simulink model "TST_CrCtl_StM"  (R2016b)
settings: Solver=FixedStepDiscrete  StartTime=0.0  StopTime=simTime  FixedStep=sampleTime  RelTol=1e-3
values from neighbouring files (symbols this model uses):
  testCase = 1    [initTST_CrCtl_StM_001.m]    (also in initTST_CrCtl_StM_002.m = 2)
libraries: simulink x31, UnitTest_Lib x18
(part 1 of 2)
settings Model: Creator=shiliwei  LastModifiedBy=shiliwei
settings DebuggingCC: SignalRangeChecking=error

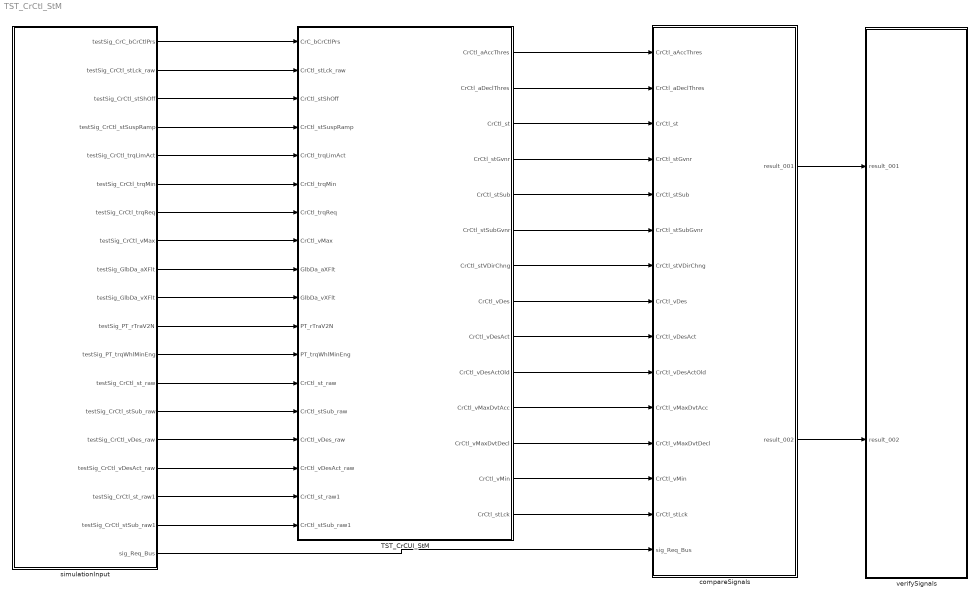
== system TST_CrCtl_StM ==
  TST_CrCUI_StM : Subsystem
  compareSignals : Subsystem
  simulationInput : Subsystem
  verifySignals : Subsystem
  wires:
  simulationInput/1(testSig_CrC_bCrCtlPrs) -> TST_CrCUI_StM/1(CrC_bCrCtlPrs)
  simulationInput/2(testSig_CrCtl_stLck_raw) -> TST_CrCUI_StM/2(CrCtl_stLck_raw)
  simulationInput/3(testSig_CrCtl_stShOff) -> TST_CrCUI_StM/3(CrCtl_stShOff)
  simulationInput/4(testSig_CrCtl_stSuspRamp) -> TST_CrCUI_StM/4(CrCtl_stSuspRamp)
  simulationInput/5(testSig_CrCtl_trqLimAct) -> TST_CrCUI_StM/5(CrCtl_trqLimAct)
  simulationInput/6(testSig_CrCtl_trqMin) -> TST_CrCUI_StM/6(CrCtl_trqMin)
  simulationInput/7(testSig_CrCtl_trqReq) -> TST_CrCUI_StM/7(CrCtl_trqReq)
  simulationInput/8(testSig_CrCtl_vMax) -> TST_CrCUI_StM/8(CrCtl_vMax)
  simulationInput/9(testSig_GlbDa_aXFlt) -> TST_CrCUI_StM/9(GlbDa_aXFlt)
  simulationInput/10(testSig_GlbDa_vXFlt) -> TST_CrCUI_StM/10(GlbDa_vXFlt)
  simulationInput/11(testSig_PT_rTraV2N) -> TST_CrCUI_StM/11(PT_rTraV2N)
  simulationInput/12(testSig_PT_trqWhlMinEng) -> TST_CrCUI_StM/12(PT_trqWhlMinEng)
  simulationInput/13(testSig_CrCtl_st_raw) -> TST_CrCUI_StM/13(CrCtl_st_raw)
  simulationInput/14(testSig_CrCtl_stSub_raw) -> TST_CrCUI_StM/14(CrCtl_stSub_raw)
  simulationInput/15(testSig_CrCtl_vDes_raw) -> TST_CrCUI_StM/15(CrCtl_vDes_raw)
  simulationInput/16(testSig_CrCtl_vDesAct_raw) -> TST_CrCUI_StM/16(CrCtl_vDesAct_raw)
  simulationInput/17(testSig_CrCtl_st_raw1) -> TST_CrCUI_StM/17(CrCtl_st_raw1)
  simulationInput/18(testSig_CrCtl_stSub_raw1) -> TST_CrCUI_StM/18(CrCtl_stSub_raw1)
  TST_CrCUI_StM/1(CrCtl_aAccThres) -> compareSignals/1(CrCtl_aAccThres)
  TST_CrCUI_StM/2(CrCtl_aDeclThres) -> compareSignals/2(CrCtl_aDeclThres)
  TST_CrCUI_StM/3(CrCtl_st) -> compareSignals/3(CrCtl_st)
  TST_CrCUI_StM/4(CrCtl_stGvnr) -> compareSignals/4(CrCtl_stGvnr)
  TST_CrCUI_StM/5(CrCtl_stSub) -> compareSignals/5(CrCtl_stSub)
  TST_CrCUI_StM/6(CrCtl_stSubGvnr) -> compareSignals/6(CrCtl_stSubGvnr)
  TST_CrCUI_StM/7(CrCtl_stVDirChng) -> compareSignals/7(CrCtl_stVDirChng)
  TST_CrCUI_StM/8(CrCtl_vDes) -> compareSignals/8(CrCtl_vDes)
  TST_CrCUI_StM/9(CrCtl_vDesAct) -> compareSignals/9(CrCtl_vDesAct)
  TST_CrCUI_StM/10(CrCtl_vDesActOld) -> compareSignals/10(CrCtl_vDesActOld)
  TST_CrCUI_StM/11(CrCtl_vMaxDvtAcc) -> compareSignals/11(CrCtl_vMaxDvtAcc)
  TST_CrCUI_StM/12(CrCtl_vMaxDvtDecl) -> compareSignals/12(CrCtl_vMaxDvtDecl)
  TST_CrCUI_StM/13(CrCtl_vMin) -> compareSignals/13(CrCtl_vMin)
  TST_CrCUI_StM/14(CrCtl_stLck) -> compareSignals/14(CrCtl_stLck)
  simulationInput/19(sig_Req_Bus) -> compareSignals/15(sig_Req_Bus)
  compareSignals/1(result_001) -> verifySignals/1(result_001)
  compareSignals/2(result_002) -> verifySignals/2(result_002)

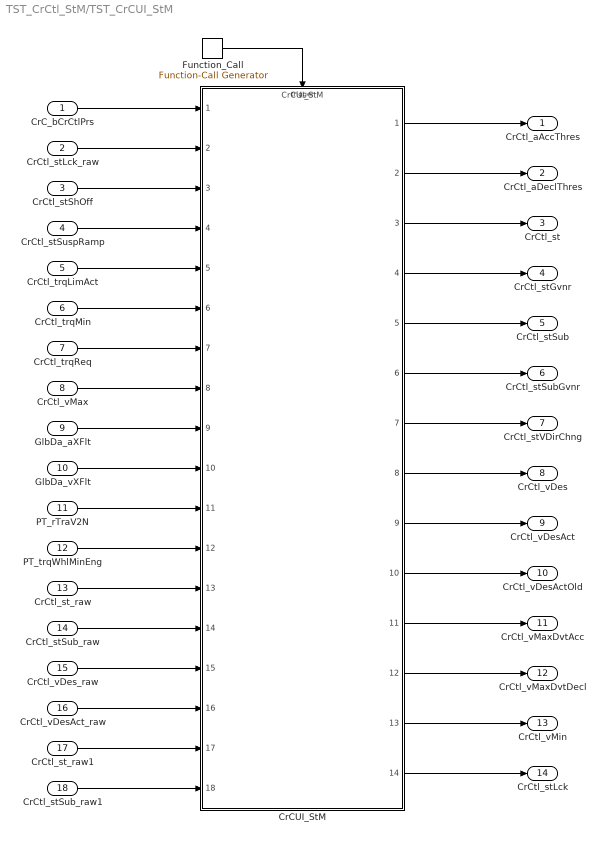
== system TST_CrCtl_StM/TST_CrCUI_StM ==
  CrC_bCrCtlPrs : Inport
  CrCtl_stLck_raw : Inport  Port=2
  CrCtl_stShOff : Inport  Port=3
  CrCtl_stSuspRamp : Inport  Port=4
  CrCtl_trqLimAct : Inport  Port=5
  CrCtl_trqMin : Inport  Port=6
  CrCtl_trqReq : Inport  Port=7
  CrCtl_vMax : Inport  Port=8
  GlbDa_aXFlt : Inport  Port=9
  GlbDa_vXFlt : Inport  Port=10
  PT_rTraV2N : Inport  Port=11
  PT_trqWhlMinEng : Inport  Port=12
  CrCtl_st_raw : Inport  Port=13
  CrCtl_stSub_raw : Inport  Port=14
  CrCtl_vDes_raw : Inport  Port=15
  CrCtl_vDesAct_raw : Inport  Port=16
  CrCtl_st_raw1 : Inport  Port=17
  CrCtl_stSub_raw1 : Inport  Port=18
  CrCUI_StM : ModelReference  ModelNameDialog=CrCUI_StM  SimulationMode=Normal  ModelReferenceVersion=1.63  TriggerPortName=function  TriggerPortTriggerType=function-call  TriggerPortStatesWhenEnabling=held
  Function_Call : simulink/Ports & Subsystems/Function-Call Generator  sample_time=sampleTime  numberOfIterations=1
  CrCtl_aAccThres : Outport
  CrCtl_aDeclThres : Outport  Port=2
  CrCtl_st : Outport  Port=3
  CrCtl_stGvnr : Outport  Port=4
  CrCtl_stSub : Outport  Port=5
  CrCtl_stSubGvnr : Outport  Port=6
  CrCtl_stVDirChng : Outport  Port=7
  CrCtl_vDes : Outport  Port=8
  CrCtl_vDesAct : Outport  Port=9
  CrCtl_vDesActOld : Outport  Port=10
  CrCtl_vMaxDvtAcc : Outport  Port=11
  CrCtl_vMaxDvtDecl : Outport  Port=12
  CrCtl_vMin : Outport  Port=13
  CrCtl_stLck : Outport  Port=14
  wires:
  Function_Call/1 -> CrCUI_StM/Trigger
  CrC_bCrCtlPrs/1 -> CrCUI_StM/1
  CrCtl_stLck_raw/1 -> CrCUI_StM/2
  CrCtl_stShOff/1 -> CrCUI_StM/3
  CrCtl_stSuspRamp/1 -> CrCUI_StM/4
  CrCtl_trqLimAct/1 -> CrCUI_StM/5
  CrCtl_trqMin/1 -> CrCUI_StM/6
  CrCtl_trqReq/1 -> CrCUI_StM/7
  CrCtl_vMax/1 -> CrCUI_StM/8
  GlbDa_aXFlt/1 -> CrCUI_StM/9
  GlbDa_vXFlt/1 -> CrCUI_StM/10
  PT_rTraV2N/1 -> CrCUI_StM/11
  PT_trqWhlMinEng/1 -> CrCUI_StM/12
  CrCtl_st_raw/1 -> CrCUI_StM/13
  CrCtl_stSub_raw/1 -> CrCUI_StM/14
  CrCtl_vDes_raw/1 -> CrCUI_StM/15
  CrCtl_vDesAct_raw/1 -> CrCUI_StM/16
  CrCtl_st_raw1/1 -> CrCUI_StM/17
  CrCtl_stSub_raw1/1 -> CrCUI_StM/18
  CrCUI_StM/1 -> CrCtl_aAccThres/1
  CrCUI_StM/2 -> CrCtl_aDeclThres/1
  CrCUI_StM/3 -> CrCtl_st/1
  CrCUI_StM/4 -> CrCtl_stGvnr/1
  CrCUI_StM/5 -> CrCtl_stSub/1
  CrCUI_StM/6 -> CrCtl_stSubGvnr/1
  CrCUI_StM/7 -> CrCtl_stVDirChng/1
  CrCUI_StM/8 -> CrCtl_vDes/1
  CrCUI_StM/9 -> CrCtl_vDesAct/1
  CrCUI_StM/10 -> CrCtl_vDesActOld/1
  CrCUI_StM/11 -> CrCtl_vMaxDvtAcc/1
  CrCUI_StM/12 -> CrCtl_vMaxDvtDecl/1
  CrCUI_StM/13 -> CrCtl_vMin/1
  CrCUI_StM/14 -> CrCtl_stLck/1

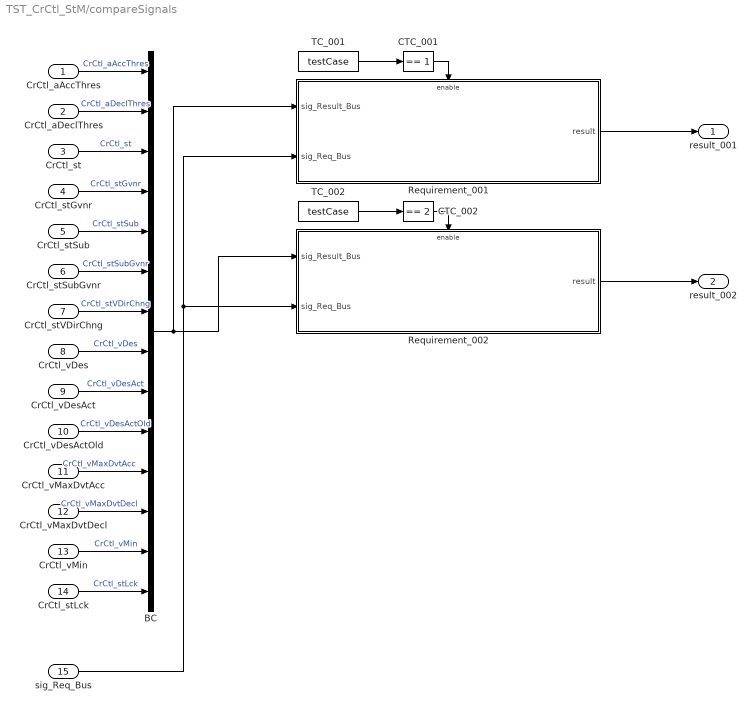
== system TST_CrCtl_StM/compareSignals ==
  CrCtl_aAccThres : Inport
  CrCtl_aDeclThres : Inport  Port=2
  CrCtl_st : Inport  Port=3
  CrCtl_stGvnr : Inport  Port=4
  CrCtl_stSub : Inport  Port=5
  CrCtl_stSubGvnr : Inport  Port=6
  CrCtl_stVDirChng : Inport  Port=7
  CrCtl_vDes : Inport  Port=8
  CrCtl_vDesAct : Inport  Port=9
  CrCtl_vDesActOld : Inport  Port=10
  CrCtl_vMaxDvtAcc : Inport  Port=11
  CrCtl_vMaxDvtDecl : Inport  Port=12
  CrCtl_vMin : Inport  Port=13
  CrCtl_stLck : Inport  Port=14
  sig_Req_Bus : Inport  Port=15
  BC : BusCreator  Inputs=14
  CTC_001 : simulink/Logic and Bit Operations/Compare To Constant  relop===  const=1  OutDataTypeStr=boolean
  CTC_002 : simulink/Logic and Bit Operations/Compare To Constant  relop===  const=2  OutDataTypeStr=boolean
  Requirement_001 : Subsystem
  Requirement_002 : Subsystem
  TC_001 : Constant  Value=testCase
  TC_002 : Constant  Value=testCase
  result_001 : Outport
  result_002 : Outport  Port=2
  wires:
  CrCtl_aAccThres/1 -> BC/1  "CrCtl_aAccThres"
  CrCtl_aDeclThres/1 -> BC/2  "CrCtl_aDeclThres"
  CrCtl_st/1 -> BC/3  "CrCtl_st"
  CrCtl_stGvnr/1 -> BC/4  "CrCtl_stGvnr"
  CrCtl_stSub/1 -> BC/5  "CrCtl_stSub"
  CrCtl_stSubGvnr/1 -> BC/6  "CrCtl_stSubGvnr"
  CrCtl_stVDirChng/1 -> BC/7  "CrCtl_stVDirChng"
  CrCtl_vDes/1 -> BC/8  "CrCtl_vDes"
  CrCtl_vDesAct/1 -> BC/9  "CrCtl_vDesAct"
  CrCtl_vDesActOld/1 -> BC/10  "CrCtl_vDesActOld"
  CrCtl_vMaxDvtAcc/1 -> BC/11  "CrCtl_vMaxDvtAcc"
  CrCtl_vMaxDvtDecl/1 -> BC/12  "CrCtl_vMaxDvtDecl"
  CrCtl_vMin/1 -> BC/13  "CrCtl_vMin"
  CrCtl_stLck/1 -> BC/14  "CrCtl_stLck"
  TC_001/1 -> CTC_001/1
  CTC_001/1 -> Requirement_001/Enable
  sig_Req_Bus/1 -> Requirement_001/2(sig_Req_Bus), Requirement_002/2(sig_Req_Bus)
  BC/1 -> Requirement_001/1(sig_Result_Bus), Requirement_002/1(sig_Result_Bus)
  Requirement_001/1(result) -> result_001/1
  TC_002/1 -> CTC_002/1
  CTC_002/1 -> Requirement_002/Enable
  Requirement_002/1(result) -> result_002/1

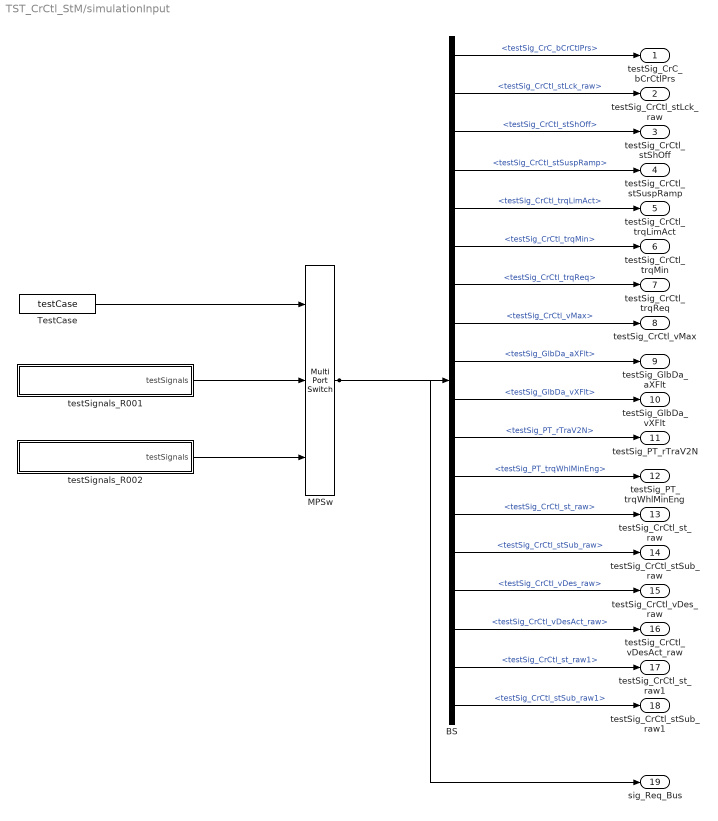
== system TST_CrCtl_StM/simulationInput ==
  BS : BusSelector  OutputSignals=testSig_CrC_bCrCtlPrs,testSig_CrCtl_stLck_raw,testSig_CrCtl_stShOff,testSig_CrCtl_stSuspRamp,testSig_CrCtl_trqLimAct,testSig_CrCtl_trqMin,testSig_CrCtl_trqReq,testSig_CrCtl_vMax,testSig_GlbDa_aXFlt,testSig_GlbDa_vXFlt,testSig_PT_rTraV2N,testSig_PT_trqWhlMinEng,testSig_CrCtl_st_raw,testSig_CrCtl_stSub_raw,testSig_CrCtl_vDes_raw,testSig_CrCtl_vDesAct_raw,testSig_CrCtl_st_raw1,testSig_CrCtl_stSub_raw1
  MPSw : MultiPortSwitch  Inputs=2  SaturateOnIntegerOverflow=on  InputSameDT=on
  TestCase : Constant  Value=testCase
  testSignals_R001 : Subsystem
  testSignals_R002 : Subsystem
  testSig_CrC_bCrCtlPrs : Outport
  testSig_CrCtl_stLck_raw : Outport  Port=2
  testSig_CrCtl_stShOff : Outport  Port=3
  testSig_CrCtl_stSuspRamp : Outport  Port=4
  testSig_CrCtl_trqLimAct : Outport  Port=5
  testSig_CrCtl_trqMin : Outport  Port=6
  testSig_CrCtl_trqReq : Outport  Port=7
  testSig_CrCtl_vMax : Outport  Port=8
  testSig_GlbDa_aXFlt : Outport  Port=9
  testSig_GlbDa_vXFlt : Outport  Port=10
  testSig_PT_rTraV2N : Outport  Port=11
  testSig_PT_trqWhlMinEng : Outport  Port=12
  testSig_CrCtl_st_raw : Outport  Port=13
  testSig_CrCtl_stSub_raw : Outport  Port=14
  testSig_CrCtl_vDes_raw : Outport  Port=15
  testSig_CrCtl_vDesAct_raw : Outport  Port=16
  testSig_CrCtl_st_raw1 : Outport  Port=17
  testSig_CrCtl_stSub_raw1 : Outport  Port=18
  sig_Req_Bus : Outport  Port=19
  wires:
  BS/1 -> testSig_CrC_bCrCtlPrs/1  "<testSig_CrC_bCrCtlPrs>"
  BS/2 -> testSig_CrCtl_stLck_raw/1  "<testSig_CrCtl_stLck_raw>"
  BS/3 -> testSig_CrCtl_stShOff/1  "<testSig_CrCtl_stShOff>"
  BS/4 -> testSig_CrCtl_stSuspRamp/1  "<testSig_CrCtl_stSuspRamp>"
  BS/5 -> testSig_CrCtl_trqLimAct/1  "<testSig_CrCtl_trqLimAct>"
  BS/6 -> testSig_CrCtl_trqMin/1  "<testSig_CrCtl_trqMin>"
  BS/7 -> testSig_CrCtl_trqReq/1  "<testSig_CrCtl_trqReq>"
  BS/8 -> testSig_CrCtl_vMax/1  "<testSig_CrCtl_vMax>"
  BS/9 -> testSig_GlbDa_aXFlt/1  "<testSig_GlbDa_aXFlt>"
  BS/10 -> testSig_GlbDa_vXFlt/1  "<testSig_GlbDa_vXFlt>"
  BS/11 -> testSig_PT_rTraV2N/1  "<testSig_PT_rTraV2N>"
  BS/12 -> testSig_PT_trqWhlMinEng/1  "<testSig_PT_trqWhlMinEng>"
  BS/13 -> testSig_CrCtl_st_raw/1  "<testSig_CrCtl_st_raw>"
  BS/14 -> testSig_CrCtl_stSub_raw/1  "<testSig_CrCtl_stSub_raw>"
  BS/15 -> testSig_CrCtl_vDes_raw/1  "<testSig_CrCtl_vDes_raw>"
  BS/16 -> testSig_CrCtl_vDesAct_raw/1  "<testSig_CrCtl_vDesAct_raw>"
  BS/17 -> testSig_CrCtl_st_raw1/1  "<testSig_CrCtl_st_raw1>"
  BS/18 -> testSig_CrCtl_stSub_raw1/1  "<testSig_CrCtl_stSub_raw1>"
  MPSw/1 -> BS/1, sig_Req_Bus/1
  TestCase/1 -> MPSw/1
  testSignals_R001/1(testSignals) -> MPSw/2
  testSignals_R002/1(testSignals) -> MPSw/3

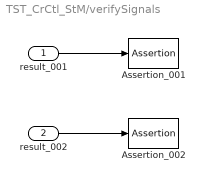
== system TST_CrCtl_StM/verifySignals ==
  result_001 : Inport
  result_002 : Inport  Port=2
  Assertion_001 : Assertion  Enabled=off
  Assertion_002 : Assertion  Enabled=off
  wires:
  result_001/1 -> Assertion_001/1
  result_002/1 -> Assertion_002/1

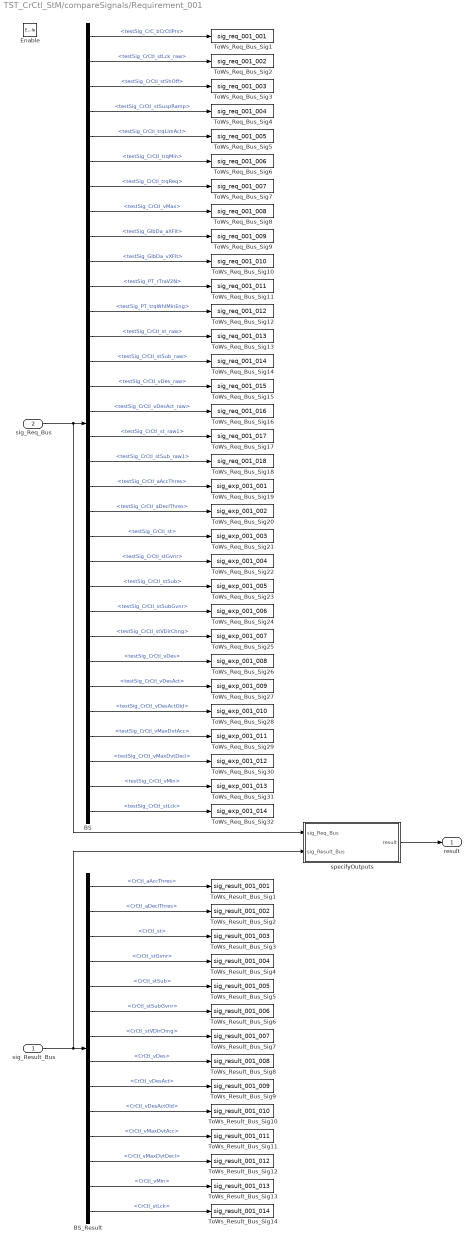
== system TST_CrCtl_StM/compareSignals/Requirement_001 ==
  sig_Result_Bus : Inport
  sig_Req_Bus : Inport  Port=2
  Enable : EnablePort
  BS : BusSelector  OutputSignals=testSig_CrC_bCrCtlPrs,testSig_CrCtl_stLck_raw,testSig_CrCtl_stShOff,testSig_CrCtl_stSuspRamp,testSig_CrCtl_trqLimAct,testSig_CrCtl_trqMin,testSig_CrCtl_trqReq,testSig_CrCtl_vMax,testSig_GlbDa_aXFlt,testSig_GlbDa_vXFlt,testSig_PT_rTraV2N,testSig_PT_trqWhlMinEng,testSig_CrCtl_st_raw,testSig_CrCtl_stSub_raw,testSig_CrCtl_vDes_raw,testSig_CrCtl_vDesAct_raw,testSig_CrCtl_st_raw1,testSig_CrCtl_stSub_raw1,testSig_CrCtl_aAccThres,testSig_CrCtl_aDeclThres,testSig_CrCtl_st,testSig_CrCtl_stGvnr,testSig_CrCtl_stSub,testSig_CrCtl_stSubGvnr,testSig_CrCtl_stVDirChng,testSig_CrCtl_vDes,testSig_CrCtl_vDesAct,testSig_CrCtl_vDesActOld,testSig_CrCtl_vMaxDvtAcc,testSig_CrCtl_vMaxDvtDecl,testSig_CrCtl_vMin,testSig_CrCtl_stLck
  BS_Result : BusSelector  OutputSignals=CrCtl_aAccThres,CrCtl_aDeclThres,CrCtl_st,CrCtl_stGvnr,CrCtl_stSub,CrCtl_stSubGvnr,CrCtl_stVDirChng,CrCtl_vDes,CrCtl_vDesAct,CrCtl_vDesActOld,CrCtl_vMaxDvtAcc,CrCtl_vMaxDvtDecl,CrCtl_vMin,CrCtl_stLck
  ToWs_Req_Bus_Sig1 : ToWorkspace  VariableName=sig_req_001_001  SaveFormat=Structure With Time
  ToWs_Req_Bus_Sig10 : ToWorkspace  VariableName=sig_req_001_010  SaveFormat=Structure With Time
  ToWs_Req_Bus_Sig11 : ToWorkspace  VariableName=sig_req_001_011  SaveFormat=Structure With Time
  ToWs_Req_Bus_Sig12 : ToWorkspace  VariableName=sig_req_001_012  SaveFormat=Structure With Time
  ToWs_Req_Bus_Sig13 : ToWorkspace  VariableName=sig_req_001_013  SaveFormat=Structure With Time
  ToWs_Req_Bus_Sig14 : ToWorkspace  VariableName=sig_req_001_014  SaveFormat=Structure With Time
  ToWs_Req_Bus_Sig15 : ToWorkspace  VariableName=sig_req_001_015  SaveFormat=Structure With Time
  ToWs_Req_Bus_Sig16 : ToWorkspace  VariableName=sig_req_001_016  SaveFormat=Structure With Time
  ToWs_Req_Bus_Sig17 : ToWorkspace  VariableName=sig_req_001_017  SaveFormat=Structure With Time
  ToWs_Req_Bus_Sig18 : ToWorkspace  VariableName=sig_req_001_018  SaveFormat=Structure With Time
  ToWs_Req_Bus_Sig19 : ToWorkspace  VariableName=sig_exp_001_001  SaveFormat=Structure With Time
  ToWs_Req_Bus_Sig2 : ToWorkspace  VariableName=sig_req_001_002  SaveFormat=Structure With Time
  ToWs_Req_Bus_Sig20 : ToWorkspace  VariableName=sig_exp_001_002  SaveFormat=Structure With Time
  ToWs_Req_Bus_Sig21 : ToWorkspace  VariableName=sig_exp_001_003  SaveFormat=Structure With Time
  ToWs_Req_Bus_Sig22 : ToWorkspace  VariableName=sig_exp_001_004  SaveFormat=Structure With Time
  ToWs_Req_Bus_Sig23 : ToWorkspace  VariableName=sig_exp_001_005  SaveFormat=Structure With Time
  ToWs_Req_Bus_Sig24 : ToWorkspace  VariableName=sig_exp_001_006  SaveFormat=Structure With Time
  ToWs_Req_Bus_Sig25 : ToWorkspace  VariableName=sig_exp_001_007  SaveFormat=Structure With Time
  ToWs_Req_Bus_Sig26 : ToWorkspace  VariableName=sig_exp_001_008  SaveFormat=Structure With Time
  ToWs_Req_Bus_Sig27 : ToWorkspace  VariableName=sig_exp_001_009  SaveFormat=Structure With Time
  ToWs_Req_Bus_Sig28 : ToWorkspace  VariableName=sig_exp_001_010  SaveFormat=Structure With Time
  ToWs_Req_Bus_Sig29 : ToWorkspace  VariableName=sig_exp_001_011  SaveFormat=Structure With Time
  ToWs_Req_Bus_Sig3 : ToWorkspace  VariableName=sig_req_001_003  SaveFormat=Structure With Time
  ToWs_Req_Bus_Sig30 : ToWorkspace  VariableName=sig_exp_001_012  SaveFormat=Structure With Time
  ToWs_Req_Bus_Sig31 : ToWorkspace  VariableName=sig_exp_001_013  SaveFormat=Structure With Time
  ToWs_Req_Bus_Sig32 : ToWorkspace  VariableName=sig_exp_001_014  SaveFormat=Structure With Time
  ToWs_Req_Bus_Sig4 : ToWorkspace  VariableName=sig_req_001_004  SaveFormat=Structure With Time
  ToWs_Req_Bus_Sig5 : ToWorkspace  VariableName=sig_req_001_005  SaveFormat=Structure With Time
  ToWs_Req_Bus_Sig6 : ToWorkspace  VariableName=sig_req_001_006  SaveFormat=Structure With Time
  ToWs_Req_Bus_Sig7 : ToWorkspace  VariableName=sig_req_001_007  SaveFormat=Structure With Time
  ToWs_Req_Bus_Sig8 : ToWorkspace  VariableName=sig_req_001_008  SaveFormat=Structure With Time
  ToWs_Req_Bus_Sig9 : ToWorkspace  VariableName=sig_req_001_009  SaveFormat=Structure With Time
  ToWs_Result_Bus_Sig1 : ToWorkspace  VariableName=sig_result_001_001  SaveFormat=Structure With Time
  ToWs_Result_Bus_Sig10 : ToWorkspace  VariableName=sig_result_001_010  SaveFormat=Structure With Time
  ToWs_Result_Bus_Sig11 : ToWorkspace  VariableName=sig_result_001_011  SaveFormat=Structure With Time
  ToWs_Result_Bus_Sig12 : ToWorkspace  VariableName=sig_result_001_012  SaveFormat=Structure With Time
  ToWs_Result_Bus_Sig13 : ToWorkspace  VariableName=sig_result_001_013  SaveFormat=Structure With Time
  ToWs_Result_Bus_Sig14 : ToWorkspace  VariableName=sig_result_001_014  SaveFormat=Structure With Time
  ToWs_Result_Bus_Sig2 : ToWorkspace  VariableName=sig_result_001_002  SaveFormat=Structure With Time
  ToWs_Result_Bus_Sig3 : ToWorkspace  VariableName=sig_result_001_003  SaveFormat=Structure With Time
  ToWs_Result_Bus_Sig4 : ToWorkspace  VariableName=sig_result_001_004  SaveFormat=Structure With Time
  ToWs_Result_Bus_Sig5 : ToWorkspace  VariableName=sig_result_001_005  SaveFormat=Structure With Time
  ToWs_Result_Bus_Sig6 : ToWorkspace  VariableName=sig_result_001_006  SaveFormat=Structure With Time
  ToWs_Result_Bus_Sig7 : ToWorkspace  VariableName=sig_result_001_007  SaveFormat=Structure With Time
  ToWs_Result_Bus_Sig8 : ToWorkspace  VariableName=sig_result_001_008  SaveFormat=Structure With Time
  ToWs_Result_Bus_Sig9 : ToWorkspace  VariableName=sig_result_001_009  SaveFormat=Structure With Time
  specifyOutputs : Subsystem
  result : Outport
  wires:
  sig_Req_Bus/1 -> BS/1, specifyOutputs/1(sig_Req_Bus)
  BS/1 -> ToWs_Req_Bus_Sig1/1  "<testSig_CrC_bCrCtlPrs>"
  BS/2 -> ToWs_Req_Bus_Sig2/1  "<testSig_CrCtl_stLck_raw>"
  BS/3 -> ToWs_Req_Bus_Sig3/1  "<testSig_CrCtl_stShOff>"
  BS/4 -> ToWs_Req_Bus_Sig4/1  "<testSig_CrCtl_stSuspRamp>"
  BS/5 -> ToWs_Req_Bus_Sig5/1  "<testSig_CrCtl_trqLimAct>"
  BS/6 -> ToWs_Req_Bus_Sig6/1  "<testSig_CrCtl_trqMin>"
  BS/7 -> ToWs_Req_Bus_Sig7/1  "<testSig_CrCtl_trqReq>"
  BS/8 -> ToWs_Req_Bus_Sig8/1  "<testSig_CrCtl_vMax>"
  BS/9 -> ToWs_Req_Bus_Sig9/1  "<testSig_GlbDa_aXFlt>"
  BS/10 -> ToWs_Req_Bus_Sig10/1  "<testSig_GlbDa_vXFlt>"
  BS/11 -> ToWs_Req_Bus_Sig11/1  "<testSig_PT_rTraV2N>"
  BS/12 -> ToWs_Req_Bus_Sig12/1  "<testSig_PT_trqWhlMinEng>"
  BS/13 -> ToWs_Req_Bus_Sig13/1  "<testSig_CrCtl_st_raw>"
  BS/14 -> ToWs_Req_Bus_Sig14/1  "<testSig_CrCtl_stSub_raw>"
  BS/15 -> ToWs_Req_Bus_Sig15/1  "<testSig_CrCtl_vDes_raw>"
  BS/16 -> ToWs_Req_Bus_Sig16/1  "<testSig_CrCtl_vDesAct_raw>"
  BS/17 -> ToWs_Req_Bus_Sig17/1  "<testSig_CrCtl_st_raw1>"
  BS/18 -> ToWs_Req_Bus_Sig18/1  "<testSig_CrCtl_stSub_raw1>"
  BS/19 -> ToWs_Req_Bus_Sig19/1  "<testSig_CrCtl_aAccThres>"
  BS/20 -> ToWs_Req_Bus_Sig20/1  "<testSig_CrCtl_aDeclThres>"
  BS/21 -> ToWs_Req_Bus_Sig21/1  "<testSig_CrCtl_st>"
  BS/22 -> ToWs_Req_Bus_Sig22/1  "<testSig_CrCtl_stGvnr>"
  BS/23 -> ToWs_Req_Bus_Sig23/1  "<testSig_CrCtl_stSub>"
  BS/24 -> ToWs_Req_Bus_Sig24/1  "<testSig_CrCtl_stSubGvnr>"
  BS/25 -> ToWs_Req_Bus_Sig25/1  "<testSig_CrCtl_stVDirChng>"
  BS/26 -> ToWs_Req_Bus_Sig26/1  "<testSig_CrCtl_vDes>"
  BS/27 -> ToWs_Req_Bus_Sig27/1  "<testSig_CrCtl_vDesAct>"
  BS/28 -> ToWs_Req_Bus_Sig28/1  "<testSig_CrCtl_vDesActOld>"
  BS/29 -> ToWs_Req_Bus_Sig29/1  "<testSig_CrCtl_vMaxDvtAcc>"
  BS/30 -> ToWs_Req_Bus_Sig30/1  "<testSig_CrCtl_vMaxDvtDecl>"
  BS/31 -> ToWs_Req_Bus_Sig31/1  "<testSig_CrCtl_vMin>"
  BS/32 -> ToWs_Req_Bus_Sig32/1  "<testSig_CrCtl_stLck>"
  sig_Result_Bus/1 -> BS_Result/1, specifyOutputs/2(sig_Result_Bus)
  BS_Result/1 -> ToWs_Result_Bus_Sig1/1  "<CrCtl_aAccThres>"
  BS_Result/2 -> ToWs_Result_Bus_Sig2/1  "<CrCtl_aDeclThres>"
  BS_Result/3 -> ToWs_Result_Bus_Sig3/1  "<CrCtl_st>"
  BS_Result/4 -> ToWs_Result_Bus_Sig4/1  "<CrCtl_stGvnr>"
  BS_Result/5 -> ToWs_Result_Bus_Sig5/1  "<CrCtl_stSub>"
  BS_Result/6 -> ToWs_Result_Bus_Sig6/1  "<CrCtl_stSubGvnr>"
  BS_Result/7 -> ToWs_Result_Bus_Sig7/1  "<CrCtl_stVDirChng>"
  BS_Result/8 -> ToWs_Result_Bus_Sig8/1  "<CrCtl_vDes>"
  BS_Result/9 -> ToWs_Result_Bus_Sig9/1  "<CrCtl_vDesAct>"
  BS_Result/10 -> ToWs_Result_Bus_Sig10/1  "<CrCtl_vDesActOld>"
  BS_Result/11 -> ToWs_Result_Bus_Sig11/1  "<CrCtl_vMaxDvtAcc>"
  BS_Result/12 -> ToWs_Result_Bus_Sig12/1  "<CrCtl_vMaxDvtDecl>"
  BS_Result/13 -> ToWs_Result_Bus_Sig13/1  "<CrCtl_vMin>"
  BS_Result/14 -> ToWs_Result_Bus_Sig14/1  "<CrCtl_stLck>"
  specifyOutputs/1(result) -> result/1

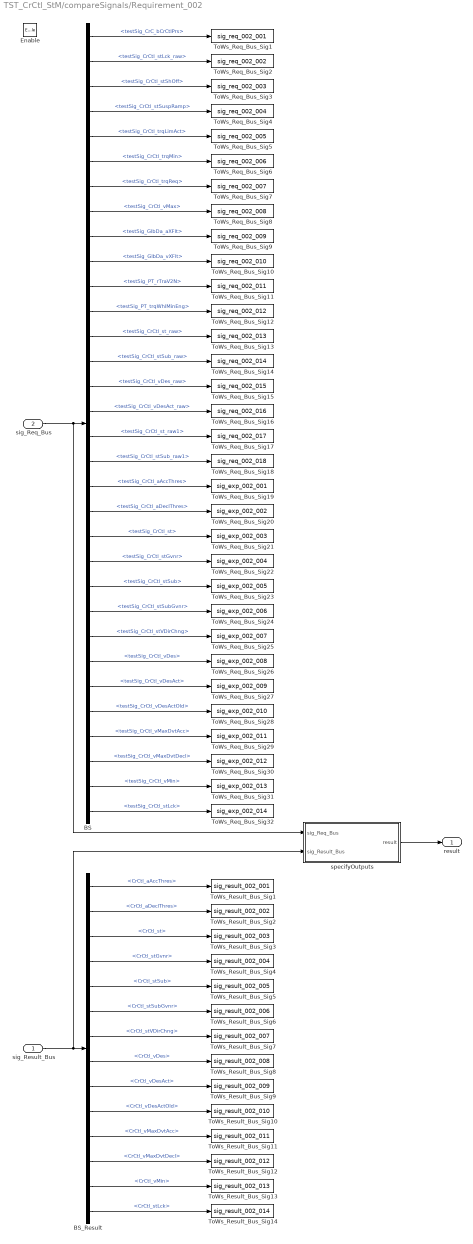
== system TST_CrCtl_StM/compareSignals/Requirement_002 ==
  sig_Result_Bus : Inport
  sig_Req_Bus : Inport  Port=2
  Enable : EnablePort
  BS : BusSelector  OutputSignals=testSig_CrC_bCrCtlPrs,testSig_CrCtl_stLck_raw,testSig_CrCtl_stShOff,testSig_CrCtl_stSuspRamp,testSig_CrCtl_trqLimAct,testSig_CrCtl_trqMin,testSig_CrCtl_trqReq,testSig_CrCtl_vMax,testSig_GlbDa_aXFlt,testSig_GlbDa_vXFlt,testSig_PT_rTraV2N,testSig_PT_trqWhlMinEng,testSig_CrCtl_st_raw,testSig_CrCtl_stSub_raw,testSig_CrCtl_vDes_raw,testSig_CrCtl_vDesAct_raw,testSig_CrCtl_st_raw1,testSig_CrCtl_stSub_raw1,testSig_CrCtl_aAccThres,testSig_CrCtl_aDeclThres,testSig_CrCtl_st,testSig_CrCtl_stGvnr,testSig_CrCtl_stSub,testSig_CrCtl_stSubGvnr,testSig_CrCtl_stVDirChng,testSig_CrCtl_vDes,testSig_CrCtl_vDesAct,testSig_CrCtl_vDesActOld,testSig_CrCtl_vMaxDvtAcc,testSig_CrCtl_vMaxDvtDecl,testSig_CrCtl_vMin,testSig_CrCtl_stLck
  BS_Result : BusSelector  OutputSignals=CrCtl_aAccThres,CrCtl_aDeclThres,CrCtl_st,CrCtl_stGvnr,CrCtl_stSub,CrCtl_stSubGvnr,CrCtl_stVDirChng,CrCtl_vDes,CrCtl_vDesAct,CrCtl_vDesActOld,CrCtl_vMaxDvtAcc,CrCtl_vMaxDvtDecl,CrCtl_vMin,CrCtl_stLck
  ToWs_Req_Bus_Sig1 : ToWorkspace  VariableName=sig_req_002_001  SaveFormat=Structure With Time
  ToWs_Req_Bus_Sig10 : ToWorkspace  VariableName=sig_req_002_010  SaveFormat=Structure With Time
  ToWs_Req_Bus_Sig11 : ToWorkspace  VariableName=sig_req_002_011  SaveFormat=Structure With Time
  ToWs_Req_Bus_Sig12 : ToWorkspace  VariableName=sig_req_002_012  SaveFormat=Structure With Time
  ToWs_Req_Bus_Sig13 : ToWorkspace  VariableName=sig_req_002_013  SaveFormat=Structure With Time
  ToWs_Req_Bus_Sig14 : ToWorkspace  VariableName=sig_req_002_014  SaveFormat=Structure With Time
  ToWs_Req_Bus_Sig15 : ToWorkspace  VariableName=sig_req_002_015  SaveFormat=Structure With Time
  ToWs_Req_Bus_Sig16 : ToWorkspace  VariableName=sig_req_002_016  SaveFormat=Structure With Time
  ToWs_Req_Bus_Sig17 : ToWorkspace  VariableName=sig_req_002_017  SaveFormat=Structure With Time
  ToWs_Req_Bus_Sig18 : ToWorkspace  VariableName=sig_req_002_018  SaveFormat=Structure With Time
  ToWs_Req_Bus_Sig19 : ToWorkspace  VariableName=sig_exp_002_001  SaveFormat=Structure With Time
  ToWs_Req_Bus_Sig2 : ToWorkspace  VariableName=sig_req_002_002  SaveFormat=Structure With Time
  ToWs_Req_Bus_Sig20 : ToWorkspace  VariableName=sig_exp_002_002  SaveFormat=Structure With Time
  ToWs_Req_Bus_Sig21 : ToWorkspace  VariableName=sig_exp_002_003  SaveFormat=Structure With Time
  ToWs_Req_Bus_Sig22 : ToWorkspace  VariableName=sig_exp_002_004  SaveFormat=Structure With Time
  ToWs_Req_Bus_Sig23 : ToWorkspace  VariableName=sig_exp_002_005  SaveFormat=Structure With Time
  ToWs_Req_Bus_Sig24 : ToWorkspace  VariableName=sig_exp_002_006  SaveFormat=Structure With Time
  ToWs_Req_Bus_Sig25 : ToWorkspace  VariableName=sig_exp_002_007  SaveFormat=Structure With Time
  ToWs_Req_Bus_Sig26 : ToWorkspace  VariableName=sig_exp_002_008  SaveFormat=Structure With Time
  ToWs_Req_Bus_Sig27 : ToWorkspace  VariableName=sig_exp_002_009  SaveFormat=Structure With Time
  ToWs_Req_Bus_Sig28 : ToWorkspace  VariableName=sig_exp_002_010  SaveFormat=Structure With Time
  ToWs_Req_Bus_Sig29 : ToWorkspace  VariableName=sig_exp_002_011  SaveFormat=Structure With Time
  ToWs_Req_Bus_Sig3 : ToWorkspace  VariableName=sig_req_002_003  SaveFormat=Structure With Time
  ToWs_Req_Bus_Sig30 : ToWorkspace  VariableName=sig_exp_002_012  SaveFormat=Structure With Time
  ToWs_Req_Bus_Sig31 : ToWorkspace  VariableName=sig_exp_002_013  SaveFormat=Structure With Time
  ToWs_Req_Bus_Sig32 : ToWorkspace  VariableName=sig_exp_002_014  SaveFormat=Structure With Time
  ToWs_Req_Bus_Sig4 : ToWorkspace  VariableName=sig_req_002_004  SaveFormat=Structure With Time
  ToWs_Req_Bus_Sig5 : ToWorkspace  VariableName=sig_req_002_005  SaveFormat=Structure With Time
  ToWs_Req_Bus_Sig6 : ToWorkspace  VariableName=sig_req_002_006  SaveFormat=Structure With Time
  ToWs_Req_Bus_Sig7 : ToWorkspace  VariableName=sig_req_002_007  SaveFormat=Structure With Time
  ToWs_Req_Bus_Sig8 : ToWorkspace  VariableName=sig_req_002_008  SaveFormat=Structure With Time
  ToWs_Req_Bus_Sig9 : ToWorkspace  VariableName=sig_req_002_009  SaveFormat=Structure With Time
  ToWs_Result_Bus_Sig1 : ToWorkspace  VariableName=sig_result_002_001  SaveFormat=Structure With Time
  ToWs_Result_Bus_Sig10 : ToWorkspace  VariableName=sig_result_002_010  SaveFormat=Structure With Time
  ToWs_Result_Bus_Sig11 : ToWorkspace  VariableName=sig_result_002_011  SaveFormat=Structure With Time
  ToWs_Result_Bus_Sig12 : ToWorkspace  VariableName=sig_result_002_012  SaveFormat=Structure With Time
  ToWs_Result_Bus_Sig13 : ToWorkspace  VariableName=sig_result_002_013  SaveFormat=Structure With Time
  ToWs_Result_Bus_Sig14 : ToWorkspace  VariableName=sig_result_002_014  SaveFormat=Structure With Time
  ToWs_Result_Bus_Sig2 : ToWorkspace  VariableName=sig_result_002_002  SaveFormat=Structure With Time
  ToWs_Result_Bus_Sig3 : ToWorkspace  VariableName=sig_result_002_003  SaveFormat=Structure With Time
  ToWs_Result_Bus_Sig4 : ToWorkspace  VariableName=sig_result_002_004  SaveFormat=Structure With Time
  ToWs_Result_Bus_Sig5 : ToWorkspace  VariableName=sig_result_002_005  SaveFormat=Structure With Time
  ToWs_Result_Bus_Sig6 : ToWorkspace  VariableName=sig_result_002_006  SaveFormat=Structure With Time
  ToWs_Result_Bus_Sig7 : ToWorkspace  VariableName=sig_result_002_007  SaveFormat=Structure With Time
  ToWs_Result_Bus_Sig8 : ToWorkspace  VariableName=sig_result_002_008  SaveFormat=Structure With Time
  ToWs_Result_Bus_Sig9 : ToWorkspace  VariableName=sig_result_002_009  SaveFormat=Structure With Time
  specifyOutputs : Subsystem
  result : Outport
  wires:
  sig_Req_Bus/1 -> BS/1, specifyOutputs/1(sig_Req_Bus)
  BS/1 -> ToWs_Req_Bus_Sig1/1  "<testSig_CrC_bCrCtlPrs>"
  BS/2 -> ToWs_Req_Bus_Sig2/1  "<testSig_CrCtl_stLck_raw>"
  BS/3 -> ToWs_Req_Bus_Sig3/1  "<testSig_CrCtl_stShOff>"
  BS/4 -> ToWs_Req_Bus_Sig4/1  "<testSig_CrCtl_stSuspRamp>"
  BS/5 -> ToWs_Req_Bus_Sig5/1  "<testSig_CrCtl_trqLimAct>"
  BS/6 -> ToWs_Req_Bus_Sig6/1  "<testSig_CrCtl_trqMin>"
  BS/7 -> ToWs_Req_Bus_Sig7/1  "<testSig_CrCtl_trqReq>"
  BS/8 -> ToWs_Req_Bus_Sig8/1  "<testSig_CrCtl_vMax>"
  BS/9 -> ToWs_Req_Bus_Sig9/1  "<testSig_GlbDa_aXFlt>"
  BS/10 -> ToWs_Req_Bus_Sig10/1  "<testSig_GlbDa_vXFlt>"
  BS/11 -> ToWs_Req_Bus_Sig11/1  "<testSig_PT_rTraV2N>"
  BS/12 -> ToWs_Req_Bus_Sig12/1  "<testSig_PT_trqWhlMinEng>"
  BS/13 -> ToWs_Req_Bus_Sig13/1  "<testSig_CrCtl_st_raw>"
  BS/14 -> ToWs_Req_Bus_Sig14/1  "<testSig_CrCtl_stSub_raw>"
  BS/15 -> ToWs_Req_Bus_Sig15/1  "<testSig_CrCtl_vDes_raw>"
  BS/16 -> ToWs_Req_Bus_Sig16/1  "<testSig_CrCtl_vDesAct_raw>"
  BS/17 -> ToWs_Req_Bus_Sig17/1  "<testSig_CrCtl_st_raw1>"
  BS/18 -> ToWs_Req_Bus_Sig18/1  "<testSig_CrCtl_stSub_raw1>"
  BS/19 -> ToWs_Req_Bus_Sig19/1  "<testSig_CrCtl_aAccThres>"
  BS/20 -> ToWs_Req_Bus_Sig20/1  "<testSig_CrCtl_aDeclThres>"
  BS/21 -> ToWs_Req_Bus_Sig21/1  "<testSig_CrCtl_st>"
  BS/22 -> ToWs_Req_Bus_Sig22/1  "<testSig_CrCtl_stGvnr>"
  BS/23 -> ToWs_Req_Bus_Sig23/1  "<testSig_CrCtl_stSub>"
  BS/24 -> ToWs_Req_Bus_Sig24/1  "<testSig_CrCtl_stSubGvnr>"
  BS/25 -> ToWs_Req_Bus_Sig25/1  "<testSig_CrCtl_stVDirChng>"
  BS/26 -> ToWs_Req_Bus_Sig26/1  "<testSig_CrCtl_vDes>"
  BS/27 -> ToWs_Req_Bus_Sig27/1  "<testSig_CrCtl_vDesAct>"
  BS/28 -> ToWs_Req_Bus_Sig28/1  "<testSig_CrCtl_vDesActOld>"
  BS/29 -> ToWs_Req_Bus_Sig29/1  "<testSig_CrCtl_vMaxDvtAcc>"
  BS/30 -> ToWs_Req_Bus_Sig30/1  "<testSig_CrCtl_vMaxDvtDecl>"
  BS/31 -> ToWs_Req_Bus_Sig31/1  "<testSig_CrCtl_vMin>"
  BS/32 -> ToWs_Req_Bus_Sig32/1  "<testSig_CrCtl_stLck>"
  sig_Result_Bus/1 -> BS_Result/1, specifyOutputs/2(sig_Result_Bus)
  BS_Result/1 -> ToWs_Result_Bus_Sig1/1  "<CrCtl_aAccThres>"
  BS_Result/2 -> ToWs_Result_Bus_Sig2/1  "<CrCtl_aDeclThres>"
  BS_Result/3 -> ToWs_Result_Bus_Sig3/1  "<CrCtl_st>"
  BS_Result/4 -> ToWs_Result_Bus_Sig4/1  "<CrCtl_stGvnr>"
  BS_Result/5 -> ToWs_Result_Bus_Sig5/1  "<CrCtl_stSub>"
  BS_Result/6 -> ToWs_Result_Bus_Sig6/1  "<CrCtl_stSubGvnr>"
  BS_Result/7 -> ToWs_Result_Bus_Sig7/1  "<CrCtl_stVDirChng>"
  BS_Result/8 -> ToWs_Result_Bus_Sig8/1  "<CrCtl_vDes>"
  BS_Result/9 -> ToWs_Result_Bus_Sig9/1  "<CrCtl_vDesAct>"
  BS_Result/10 -> ToWs_Result_Bus_Sig10/1  "<CrCtl_vDesActOld>"
  BS_Result/11 -> ToWs_Result_Bus_Sig11/1  "<CrCtl_vMaxDvtAcc>"
  BS_Result/12 -> ToWs_Result_Bus_Sig12/1  "<CrCtl_vMaxDvtDecl>"
  BS_Result/13 -> ToWs_Result_Bus_Sig13/1  "<CrCtl_vMin>"
  BS_Result/14 -> ToWs_Result_Bus_Sig14/1  "<CrCtl_stLck>"
  specifyOutputs/1(result) -> result/1

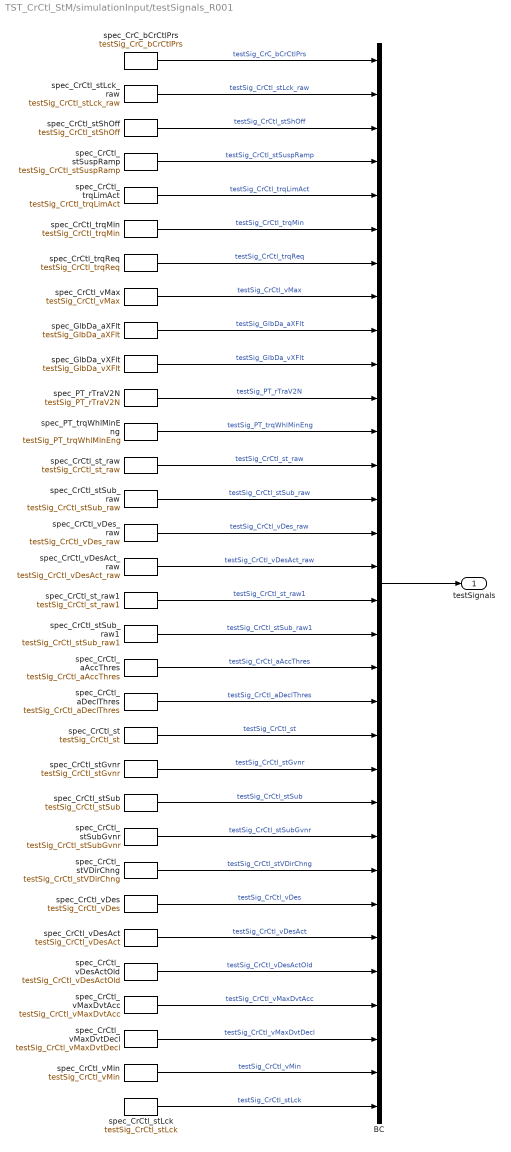
== system TST_CrCtl_StM/simulationInput/testSignals_R001 ==
  BC : BusCreator  Inputs=32
  spec_CrC_bCrCtlPrs : FromWorkspace  VariableName=testSig_CrC_bCrCtlPrs  Interpolate=off  OutputAfterFinalValue=Holding final value
  spec_CrCtl_aAccThres : FromWorkspace  VariableName=testSig_CrCtl_aAccThres  Interpolate=off  OutputAfterFinalValue=Holding final value
  spec_CrCtl_aDeclThres : FromWorkspace  VariableName=testSig_CrCtl_aDeclThres  Interpolate=off  OutputAfterFinalValue=Holding final value
  spec_CrCtl_st : FromWorkspace  VariableName=testSig_CrCtl_st  Interpolate=off  OutputAfterFinalValue=Holding final value
  spec_CrCtl_stGvnr : FromWorkspace  VariableName=testSig_CrCtl_stGvnr  Interpolate=off  OutputAfterFinalValue=Holding final value
  spec_CrCtl_stLck : FromWorkspace  VariableName=testSig_CrCtl_stLck  Interpolate=off  OutputAfterFinalValue=Holding final value
  spec_CrCtl_stLck_raw : FromWorkspace  VariableName=testSig_CrCtl_stLck_raw  Interpolate=off  OutputAfterFinalValue=Holding final value
  spec_CrCtl_stShOff : FromWorkspace  VariableName=testSig_CrCtl_stShOff  Interpolate=off  OutputAfterFinalValue=Holding final value
  spec_CrCtl_stSub : FromWorkspace  VariableName=testSig_CrCtl_stSub  Interpolate=off  OutputAfterFinalValue=Holding final value
  spec_CrCtl_stSubGvnr : FromWorkspace  VariableName=testSig_CrCtl_stSubGvnr  Interpolate=off  OutputAfterFinalValue=Holding final value
  spec_CrCtl_stSub_raw : FromWorkspace  VariableName=testSig_CrCtl_stSub_raw  Interpolate=off  OutputAfterFinalValue=Holding final value
  spec_CrCtl_stSub_raw1 : FromWorkspace  VariableName=testSig_CrCtl_stSub_raw1  Interpolate=off  OutputAfterFinalValue=Holding final value
  spec_CrCtl_stSuspRamp : FromWorkspace  VariableName=testSig_CrCtl_stSuspRamp  Interpolate=off  OutputAfterFinalValue=Holding final value
  spec_CrCtl_stVDirChng : FromWorkspace  VariableName=testSig_CrCtl_stVDirChng  Interpolate=off  OutputAfterFinalValue=Holding final value
  spec_CrCtl_st_raw : FromWorkspace  VariableName=testSig_CrCtl_st_raw  Interpolate=off  OutputAfterFinalValue=Holding final value
  spec_CrCtl_st_raw1 : FromWorkspace  VariableName=testSig_CrCtl_st_raw1  Interpolate=off  OutputAfterFinalValue=Holding final value
  spec_CrCtl_trqLimAct : FromWorkspace  VariableName=testSig_CrCtl_trqLimAct  Interpolate=off  OutputAfterFinalValue=Holding final value
  spec_CrCtl_trqMin : FromWorkspace  VariableName=testSig_CrCtl_trqMin  Interpolate=off  OutputAfterFinalValue=Holding final value
  spec_CrCtl_trqReq : FromWorkspace  VariableName=testSig_CrCtl_trqReq  Interpolate=off  OutputAfterFinalValue=Holding final value
  spec_CrCtl_vDes : FromWorkspace  VariableName=testSig_CrCtl_vDes  Interpolate=off  OutputAfterFinalValue=Holding final value
  spec_CrCtl_vDesAct : FromWorkspace  VariableName=testSig_CrCtl_vDesAct  Interpolate=off  OutputAfterFinalValue=Holding final value
  spec_CrCtl_vDesActOld : FromWorkspace  VariableName=testSig_CrCtl_vDesActOld  Interpolate=off  OutputAfterFinalValue=Holding final value
  spec_CrCtl_vDesAct_raw : FromWorkspace  VariableName=testSig_CrCtl_vDesAct_raw  Interpolate=off  OutputAfterFinalValue=Holding final value
  spec_CrCtl_vDes_raw : FromWorkspace  VariableName=testSig_CrCtl_vDes_raw  Interpolate=off  OutputAfterFinalValue=Holding final value
  spec_CrCtl_vMax : FromWorkspace  VariableName=testSig_CrCtl_vMax  Interpolate=off  OutputAfterFinalValue=Holding final value
  spec_CrCtl_vMaxDvtAcc : FromWorkspace  VariableName=testSig_CrCtl_vMaxDvtAcc  Interpolate=off  OutputAfterFinalValue=Holding final value
  spec_CrCtl_vMaxDvtDecl : FromWorkspace  VariableName=testSig_CrCtl_vMaxDvtDecl  Interpolate=off  OutputAfterFinalValue=Holding final value
  spec_CrCtl_vMin : FromWorkspace  VariableName=testSig_CrCtl_vMin  Interpolate=off  OutputAfterFinalValue=Holding final value
  spec_GlbDa_aXFlt : FromWorkspace  VariableName=testSig_GlbDa_aXFlt  Interpolate=off  OutputAfterFinalValue=Holding final value
  spec_GlbDa_vXFlt : FromWorkspace  VariableName=testSig_GlbDa_vXFlt  Interpolate=off  OutputAfterFinalValue=Holding final value
  spec_PT_rTraV2N : FromWorkspace  VariableName=testSig_PT_rTraV2N  Interpolate=off  OutputAfterFinalValue=Holding final value
  spec_PT_trqWhlMinEng : FromWorkspace  VariableName=testSig_PT_trqWhlMinEng  Interpolate=off  OutputAfterFinalValue=Holding final value
  testSignals : Outport
  wires:
  BC/1 -> testSignals/1
  spec_CrC_bCrCtlPrs/1 -> BC/1  "testSig_CrC_bCrCtlPrs"
  spec_CrCtl_stLck_raw/1 -> BC/2  "testSig_CrCtl_stLck_raw"
  spec_CrCtl_stShOff/1 -> BC/3  "testSig_CrCtl_stShOff"
  spec_CrCtl_stSuspRamp/1 -> BC/4  "testSig_CrCtl_stSuspRamp"
  spec_CrCtl_trqLimAct/1 -> BC/5  "testSig_CrCtl_trqLimAct"
  spec_CrCtl_trqMin/1 -> BC/6  "testSig_CrCtl_trqMin"
  spec_CrCtl_trqReq/1 -> BC/7  "testSig_CrCtl_trqReq"
  spec_CrCtl_vMax/1 -> BC/8  "testSig_CrCtl_vMax"
  spec_GlbDa_aXFlt/1 -> BC/9  "testSig_GlbDa_aXFlt"
  spec_GlbDa_vXFlt/1 -> BC/10  "testSig_GlbDa_vXFlt"
  spec_PT_rTraV2N/1 -> BC/11  "testSig_PT_rTraV2N"
  spec_PT_trqWhlMinEng/1 -> BC/12  "testSig_PT_trqWhlMinEng"
  spec_CrCtl_st_raw/1 -> BC/13  "testSig_CrCtl_st_raw"
  spec_CrCtl_stSub_raw/1 -> BC/14  "testSig_CrCtl_stSub_raw"
  spec_CrCtl_vDes_raw/1 -> BC/15  "testSig_CrCtl_vDes_raw"
  spec_CrCtl_vDesAct_raw/1 -> BC/16  "testSig_CrCtl_vDesAct_raw"
  spec_CrCtl_st_raw1/1 -> BC/17  "testSig_CrCtl_st_raw1"
  spec_CrCtl_stSub_raw1/1 -> BC/18  "testSig_CrCtl_stSub_raw1"
  spec_CrCtl_aAccThres/1 -> BC/19  "testSig_CrCtl_aAccThres"
  spec_CrCtl_aDeclThres/1 -> BC/20  "testSig_CrCtl_aDeclThres"
  spec_CrCtl_st/1 -> BC/21  "testSig_CrCtl_st"
  spec_CrCtl_stGvnr/1 -> BC/22  "testSig_CrCtl_stGvnr"
  spec_CrCtl_stSub/1 -> BC/23  "testSig_CrCtl_stSub"
  spec_CrCtl_stSubGvnr/1 -> BC/24  "testSig_CrCtl_stSubGvnr"
  spec_CrCtl_stVDirChng/1 -> BC/25  "testSig_CrCtl_stVDirChng"
  spec_CrCtl_vDes/1 -> BC/26  "testSig_CrCtl_vDes"
  spec_CrCtl_vDesAct/1 -> BC/27  "testSig_CrCtl_vDesAct"
  spec_CrCtl_vDesActOld/1 -> BC/28  "testSig_CrCtl_vDesActOld"
  spec_CrCtl_vMaxDvtAcc/1 -> BC/29  "testSig_CrCtl_vMaxDvtAcc"
  spec_CrCtl_vMaxDvtDecl/1 -> BC/30  "testSig_CrCtl_vMaxDvtDecl"
  spec_CrCtl_vMin/1 -> BC/31  "testSig_CrCtl_vMin"
  spec_CrCtl_stLck/1 -> BC/32  "testSig_CrCtl_stLck"

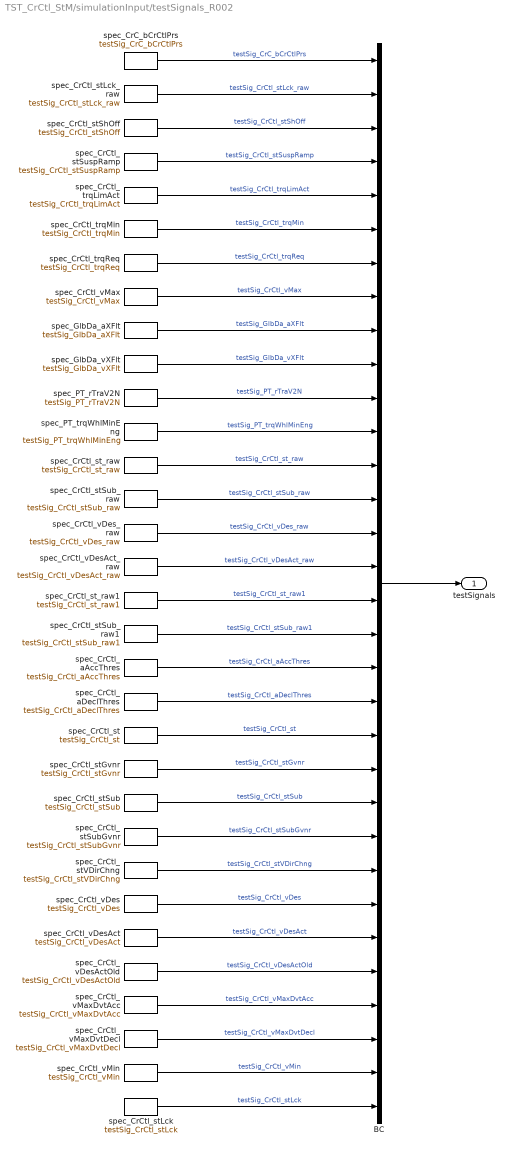
== system TST_CrCtl_StM/simulationInput/testSignals_R002 ==
  BC : BusCreator  Inputs=32
  spec_CrC_bCrCtlPrs : FromWorkspace  VariableName=testSig_CrC_bCrCtlPrs  Interpolate=off  OutputAfterFinalValue=Holding final value
  spec_CrCtl_aAccThres : FromWorkspace  VariableName=testSig_CrCtl_aAccThres  Interpolate=off  OutputAfterFinalValue=Holding final value
  spec_CrCtl_aDeclThres : FromWorkspace  VariableName=testSig_CrCtl_aDeclThres  Interpolate=off  OutputAfterFinalValue=Holding final value
  spec_CrCtl_st : FromWorkspace  VariableName=testSig_CrCtl_st  Interpolate=off  OutputAfterFinalValue=Holding final value
  spec_CrCtl_stGvnr : FromWorkspace  VariableName=testSig_CrCtl_stGvnr  Interpolate=off  OutputAfterFinalValue=Holding final value
  spec_CrCtl_stLck : FromWorkspace  VariableName=testSig_CrCtl_stLck  Interpolate=off  OutputAfterFinalValue=Holding final value
  spec_CrCtl_stLck_raw : FromWorkspace  VariableName=testSig_CrCtl_stLck_raw  Interpolate=off  OutputAfterFinalValue=Holding final value
  spec_CrCtl_stShOff : FromWorkspace  VariableName=testSig_CrCtl_stShOff  Interpolate=off  OutputAfterFinalValue=Holding final value
  spec_CrCtl_stSub : FromWorkspace  VariableName=testSig_CrCtl_stSub  Interpolate=off  OutputAfterFinalValue=Holding final value
  spec_CrCtl_stSubGvnr : FromWorkspace  VariableName=testSig_CrCtl_stSubGvnr  Interpolate=off  OutputAfterFinalValue=Holding final value
  spec_CrCtl_stSub_raw : FromWorkspace  VariableName=testSig_CrCtl_stSub_raw  Interpolate=off  OutputAfterFinalValue=Holding final value
  spec_CrCtl_stSub_raw1 : FromWorkspace  VariableName=testSig_CrCtl_stSub_raw1  Interpolate=off  OutputAfterFinalValue=Holding final value
  spec_CrCtl_stSuspRamp : FromWorkspace  VariableName=testSig_CrCtl_stSuspRamp  Interpolate=off  OutputAfterFinalValue=Holding final value
  spec_CrCtl_stVDirChng : FromWorkspace  VariableName=testSig_CrCtl_stVDirChng  Interpolate=off  OutputAfterFinalValue=Holding final value
  spec_CrCtl_st_raw : FromWorkspace  VariableName=testSig_CrCtl_st_raw  Interpolate=off  OutputAfterFinalValue=Holding final value
  spec_CrCtl_st_raw1 : FromWorkspace  VariableName=testSig_CrCtl_st_raw1  Interpolate=off  OutputAfterFinalValue=Holding final value
  spec_CrCtl_trqLimAct : FromWorkspace  VariableName=testSig_CrCtl_trqLimAct  Interpolate=off  OutputAfterFinalValue=Holding final value
  spec_CrCtl_trqMin : FromWorkspace  VariableName=testSig_CrCtl_trqMin  Interpolate=off  OutputAfterFinalValue=Holding final value
  spec_CrCtl_trqReq : FromWorkspace  VariableName=testSig_CrCtl_trqReq  Interpolate=off  OutputAfterFinalValue=Holding final value
  spec_CrCtl_vDes : FromWorkspace  VariableName=testSig_CrCtl_vDes  Interpolate=off  OutputAfterFinalValue=Holding final value
  spec_CrCtl_vDesAct : FromWorkspace  VariableName=testSig_CrCtl_vDesAct  Interpolate=off  OutputAfterFinalValue=Holding final value
  spec_CrCtl_vDesActOld : FromWorkspace  VariableName=testSig_CrCtl_vDesActOld  Interpolate=off  OutputAfterFinalValue=Holding final value
  spec_CrCtl_vDesAct_raw : FromWorkspace  VariableName=testSig_CrCtl_vDesAct_raw  Interpolate=off  OutputAfterFinalValue=Holding final value
  spec_CrCtl_vDes_raw : FromWorkspace  VariableName=testSig_CrCtl_vDes_raw  Interpolate=off  OutputAfterFinalValue=Holding final value
  spec_CrCtl_vMax : FromWorkspace  VariableName=testSig_CrCtl_vMax  Interpolate=off  OutputAfterFinalValue=Holding final value
  spec_CrCtl_vMaxDvtAcc : FromWorkspace  VariableName=testSig_CrCtl_vMaxDvtAcc  Interpolate=off  OutputAfterFinalValue=Holding final value
  spec_CrCtl_vMaxDvtDecl : FromWorkspace  VariableName=testSig_CrCtl_vMaxDvtDecl  Interpolate=off  OutputAfterFinalValue=Holding final value
  spec_CrCtl_vMin : FromWorkspace  VariableName=testSig_CrCtl_vMin  Interpolate=off  OutputAfterFinalValue=Holding final value
  spec_GlbDa_aXFlt : FromWorkspace  VariableName=testSig_GlbDa_aXFlt  Interpolate=off  OutputAfterFinalValue=Holding final value
  spec_GlbDa_vXFlt : FromWorkspace  VariableName=testSig_GlbDa_vXFlt  Interpolate=off  OutputAfterFinalValue=Holding final value
  spec_PT_rTraV2N : FromWorkspace  VariableName=testSig_PT_rTraV2N  Interpolate=off  OutputAfterFinalValue=Holding final value
  spec_PT_trqWhlMinEng : FromWorkspace  VariableName=testSig_PT_trqWhlMinEng  Interpolate=off  OutputAfterFinalValue=Holding final value
  testSignals : Outport
  wires:
  BC/1 -> testSignals/1
  spec_CrC_bCrCtlPrs/1 -> BC/1  "testSig_CrC_bCrCtlPrs"
  spec_CrCtl_stLck_raw/1 -> BC/2  "testSig_CrCtl_stLck_raw"
  spec_CrCtl_stShOff/1 -> BC/3  "testSig_CrCtl_stShOff"
  spec_CrCtl_stSuspRamp/1 -> BC/4  "testSig_CrCtl_stSuspRamp"
  spec_CrCtl_trqLimAct/1 -> BC/5  "testSig_CrCtl_trqLimAct"
  spec_CrCtl_trqMin/1 -> BC/6  "testSig_CrCtl_trqMin"
  spec_CrCtl_trqReq/1 -> BC/7  "testSig_CrCtl_trqReq"
  spec_CrCtl_vMax/1 -> BC/8  "testSig_CrCtl_vMax"
  spec_GlbDa_aXFlt/1 -> BC/9  "testSig_GlbDa_aXFlt"
  spec_GlbDa_vXFlt/1 -> BC/10  "testSig_GlbDa_vXFlt"
  spec_PT_rTraV2N/1 -> BC/11  "testSig_PT_rTraV2N"
  spec_PT_trqWhlMinEng/1 -> BC/12  "testSig_PT_trqWhlMinEng"
  spec_CrCtl_st_raw/1 -> BC/13  "testSig_CrCtl_st_raw"
  spec_CrCtl_stSub_raw/1 -> BC/14  "testSig_CrCtl_stSub_raw"
  spec_CrCtl_vDes_raw/1 -> BC/15  "testSig_CrCtl_vDes_raw"
  spec_CrCtl_vDesAct_raw/1 -> BC/16  "testSig_CrCtl_vDesAct_raw"
  spec_CrCtl_st_raw1/1 -> BC/17  "testSig_CrCtl_st_raw1"
  spec_CrCtl_stSub_raw1/1 -> BC/18  "testSig_CrCtl_stSub_raw1"
  spec_CrCtl_aAccThres/1 -> BC/19  "testSig_CrCtl_aAccThres"
  spec_CrCtl_aDeclThres/1 -> BC/20  "testSig_CrCtl_aDeclThres"
  spec_CrCtl_st/1 -> BC/21  "testSig_CrCtl_st"
  spec_CrCtl_stGvnr/1 -> BC/22  "testSig_CrCtl_stGvnr"
  spec_CrCtl_stSub/1 -> BC/23  "testSig_CrCtl_stSub"
  spec_CrCtl_stSubGvnr/1 -> BC/24  "testSig_CrCtl_stSubGvnr"
  spec_CrCtl_stVDirChng/1 -> BC/25  "testSig_CrCtl_stVDirChng"
  spec_CrCtl_vDes/1 -> BC/26  "testSig_CrCtl_vDes"
  spec_CrCtl_vDesAct/1 -> BC/27  "testSig_CrCtl_vDesAct"
  spec_CrCtl_vDesActOld/1 -> BC/28  "testSig_CrCtl_vDesActOld"
  spec_CrCtl_vMaxDvtAcc/1 -> BC/29  "testSig_CrCtl_vMaxDvtAcc"
  spec_CrCtl_vMaxDvtDecl/1 -> BC/30  "testSig_CrCtl_vMaxDvtDecl"
  spec_CrCtl_vMin/1 -> BC/31  "testSig_CrCtl_vMin"
  spec_CrCtl_stLck/1 -> BC/32  "testSig_CrCtl_stLck"

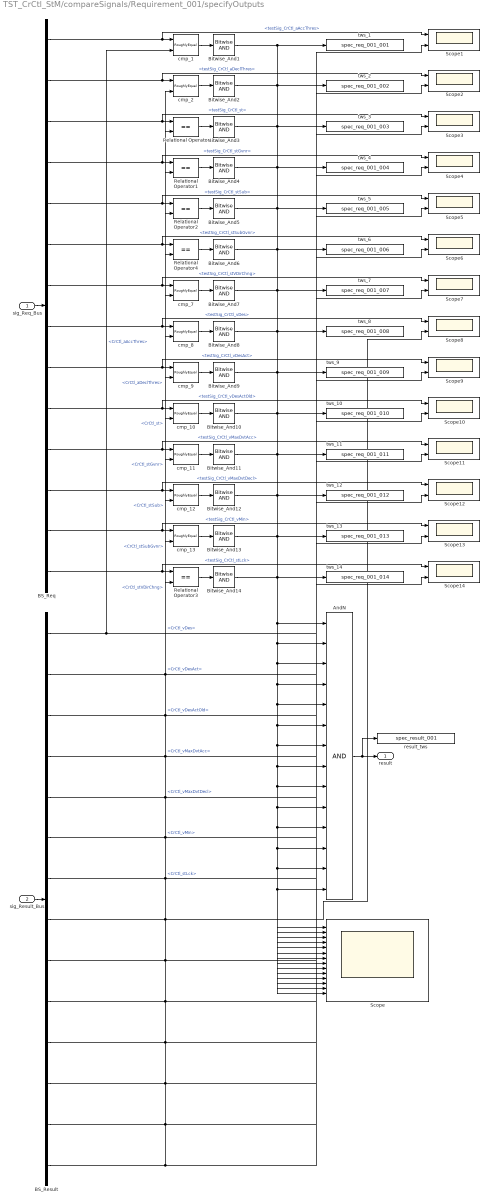
== system TST_CrCtl_StM/compareSignals/Requirement_001/specifyOutputs ==
  sig_Req_Bus : Inport
  sig_Result_Bus : Inport  Port=2
  AndN : Logic  Inputs=14
  BS_Req : BusSelector  OutputSignals=testSig_CrCtl_aAccThres,testSig_CrCtl_aDeclThres,testSig_CrCtl_st,testSig_CrCtl_stGvnr,testSig_CrCtl_stSub,testSig_CrCtl_stSubGvnr,testSig_CrCtl_stVDirChng,testSig_CrCtl_vDes,testSig_CrCtl_vDesAct,testSig_CrCtl_vDesActOld,testSig_CrCtl_vMaxDvtAcc,testSig_CrCtl_vMaxDvtDecl,testSig_CrCtl_vMin,testSig_CrCtl_stLck
  BS_Result : BusSelector  OutputSignals=CrCtl_aAccThres,CrCtl_aDeclThres,CrCtl_st,CrCtl_stGvnr,CrCtl_stSub,CrCtl_stSubGvnr,CrCtl_stVDirChng,CrCtl_vDes,CrCtl_vDesAct,CrCtl_vDesActOld,CrCtl_vMaxDvtAcc,CrCtl_vMaxDvtDecl,CrCtl_vMin,CrCtl_stLck
  Bitwise_And{1..14} (14 alike) : simulink/Logic and Bit Operations/Bitwise Operator  logicop=AND  UseBitMask=off  BitMask=bin2dec('11011001')  BitMaskRealWorld=Stored Integer
  Relational Operator{,1..4} (5 alike) : RelationalOperator  Operator===  OutDataTypeStr=boolean  RndMeth=Simplest
  Scope : Scope  NumInputPorts=14
  Scope{1..14} (14 alike) : Scope  NumInputPorts=2
  cmp_{1..2,7..13} (9 alike) : UnitTest_Lib/RoughlyEqual  slope=0.1
  result_tws : ToWorkspace  VariableName=spec_result_001
  tws_1 : ToWorkspace  VariableName=spec_req_001_001
  tws_10 : ToWorkspace  VariableName=spec_req_001_010
  tws_11 : ToWorkspace  VariableName=spec_req_001_011
  tws_12 : ToWorkspace  VariableName=spec_req_001_012
  tws_13 : ToWorkspace  VariableName=spec_req_001_013
  tws_14 : ToWorkspace  VariableName=spec_req_001_014
  tws_2 : ToWorkspace  VariableName=spec_req_001_002
  tws_3 : ToWorkspace  VariableName=spec_req_001_003
  tws_4 : ToWorkspace  VariableName=spec_req_001_004
  tws_5 : ToWorkspace  VariableName=spec_req_001_005
  tws_6 : ToWorkspace  VariableName=spec_req_001_006
  tws_7 : ToWorkspace  VariableName=spec_req_001_007
  tws_8 : ToWorkspace  VariableName=spec_req_001_008
  tws_9 : ToWorkspace  VariableName=spec_req_001_009
  result : Outport
  wires:
  sig_Req_Bus/1 -> BS_Req/1
  sig_Result_Bus/1 -> BS_Result/1
  AndN/1 -> result/1, result_tws/1
  BS_Req/1 -> cmp_1/1, Scope1/1  "<testSig_CrCtl_aAccThres>"
  BS_Result/1 -> cmp_1/2, Scope1/2  "<CrCtl_aAccThres>"
  cmp_1/1 -> Bitwise_And1/1
  Bitwise_And1/1 -> AndN/1, Scope/1, tws_1/1
  BS_Req/2 -> cmp_2/1, Scope2/1  "<testSig_CrCtl_aDeclThres>"
  BS_Result/2 -> cmp_2/2, Scope2/2  "<CrCtl_aDeclThres>"
  cmp_2/1 -> Bitwise_And2/1
  Bitwise_And2/1 -> AndN/2, Scope/2, tws_2/1
  BS_Req/3 -> Relational Operator/1, Scope3/1  "<testSig_CrCtl_st>"
  BS_Result/3 -> Relational Operator/2, Scope3/2  "<CrCtl_st>"
  Relational Operator/1 -> Bitwise_And3/1
  Bitwise_And3/1 -> AndN/3, Scope/3, tws_3/1
  BS_Req/4 -> Relational Operator1/1, Scope4/1  "<testSig_CrCtl_stGvnr>"
  BS_Result/4 -> Relational Operator1/2, Scope4/2  "<CrCtl_stGvnr>"
  Relational Operator1/1 -> Bitwise_And4/1
  Bitwise_And4/1 -> AndN/4, Scope/4, tws_4/1
  BS_Req/5 -> Relational Operator2/1, Scope5/1  "<testSig_CrCtl_stSub>"
  BS_Result/5 -> Relational Operator2/2, Scope5/2  "<CrCtl_stSub>"
  Relational Operator2/1 -> Bitwise_And5/1
  Bitwise_And5/1 -> AndN/5, Scope/5, tws_5/1
  BS_Req/6 -> Relational Operator4/1, Scope6/1  "<testSig_CrCtl_stSubGvnr>"
  BS_Result/6 -> Relational Operator4/2, Scope6/2  "<CrCtl_stSubGvnr>"
  Relational Operator4/1 -> Bitwise_And6/1
  Bitwise_And6/1 -> AndN/6, Scope/6, tws_6/1
  BS_Req/7 -> cmp_7/1, Scope7/1  "<testSig_CrCtl_stVDirChng>"
  BS_Result/7 -> cmp_7/2, Scope7/2  "<CrCtl_stVDirChng>"
  cmp_7/1 -> Bitwise_And7/1
  Bitwise_And7/1 -> AndN/7, Scope/7, tws_7/1
  BS_Req/8 -> cmp_8/1, Scope8/1  "<testSig_CrCtl_vDes>"
  BS_Result/8 -> cmp_8/2, Scope8/2  "<CrCtl_vDes>"
  cmp_8/1 -> Bitwise_And8/1
  Bitwise_And8/1 -> AndN/8, Scope/8, tws_8/1
  BS_Req/9 -> cmp_9/1, Scope9/1  "<testSig_CrCtl_vDesAct>"
  BS_Result/9 -> cmp_9/2, Scope9/2  "<CrCtl_vDesAct>"
  cmp_9/1 -> Bitwise_And9/1
  Bitwise_And9/1 -> AndN/9, Scope/9, tws_9/1
  BS_Req/10 -> cmp_10/1, Scope10/1  "<testSig_CrCtl_vDesActOld>"
  BS_Result/10 -> cmp_10/2, Scope10/2  "<CrCtl_vDesActOld>"
  cmp_10/1 -> Bitwise_And10/1
  Bitwise_And10/1 -> AndN/10, Scope/10, tws_10/1
  BS_Req/11 -> cmp_11/1, Scope11/1  "<testSig_CrCtl_vMaxDvtAcc>"
  BS_Result/11 -> cmp_11/2, Scope11/2  "<CrCtl_vMaxDvtAcc>"
  cmp_11/1 -> Bitwise_And11/1
  Bitwise_And11/1 -> AndN/11, Scope/11, tws_11/1
  BS_Req/12 -> cmp_12/1, Scope12/1  "<testSig_CrCtl_vMaxDvtDecl>"
  BS_Result/12 -> cmp_12/2, Scope12/2  "<CrCtl_vMaxDvtDecl>"
  cmp_12/1 -> Bitwise_And12/1
  Bitwise_And12/1 -> AndN/12, Scope/12, tws_12/1
  BS_Req/13 -> cmp_13/1, Scope13/1  "<testSig_CrCtl_vMin>"
  BS_Result/13 -> cmp_13/2, Scope13/2  "<CrCtl_vMin>"
  cmp_13/1 -> Bitwise_And13/1
  Bitwise_And13/1 -> AndN/13, Scope/13, tws_13/1
  BS_Req/14 -> Relational Operator3/1, Scope14/1  "<testSig_CrCtl_stLck>"
  BS_Result/14 -> Relational Operator3/2, Scope14/2  "<CrCtl_stLck>"
  Relational Operator3/1 -> Bitwise_And14/1
  Bitwise_And14/1 -> AndN/14, Scope/14, tws_14/1
